simulink model "WorkstationModel_dynamicSequencing"  (R2015b)
settings: Solver=VariableStepDiscrete  StartTime=0.0  StopTime=1000  RelTol=1e-3
undefined symbols (not defined in the file): des
settings Model: Creator=tsprock3  LastModifiedBy=tsprock3
settings SolverCC: MaxConsecutiveZCs=10000
settings DataIOCC: InitialState=state  SaveFinalState=on  SaveFormat=Array
settings HardwareCC: ProdBitPerPointer=32  ProdLargestAtomicFloat=None  ProdIntDivRoundTo=Undefined  ProdEndianess=Unspecified  ProdWordSize=32  ProdHWDeviceType=32-bit Generic
settings GRTTargetCC: GeneratePreprocessorConditionals=Disable all
settings ConfigComp: CovModelRefEnable=Off

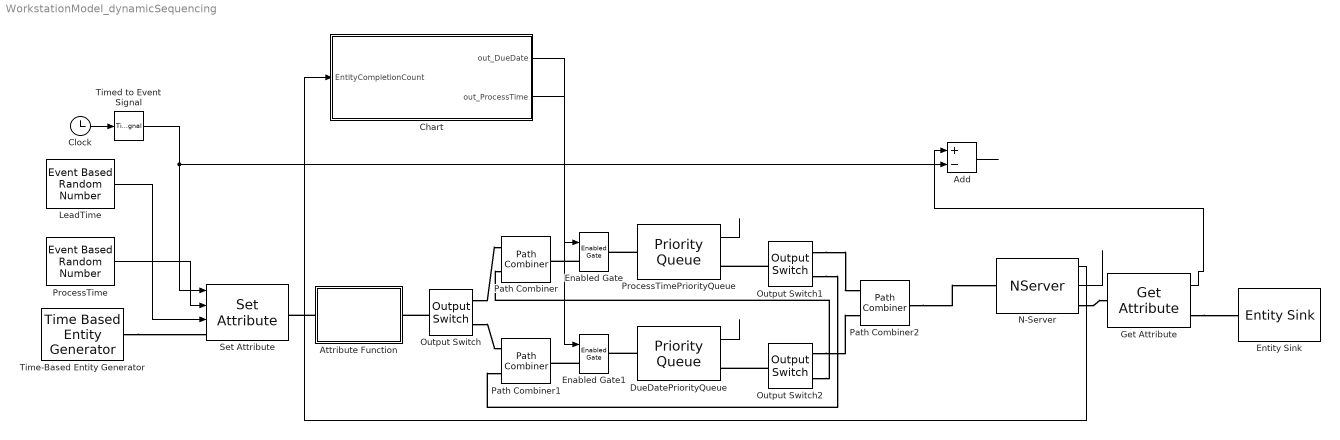
== system WorkstationModel_dynamicSequencing ==
  Add : Sum  Inputs=+-
  Attribute Function : Subsystem  LoadFcn=des.afb.attributefunction_support(gcb,'LoadFcn');  StartFcn=des.afb.attributefunction_support(gcb,'StartFcn');  mask(Attribute Function){OutputNamePrefix=out_}
      mask prompts: OutputNamePrefix "Prefix name"
      settings: CopyFcn=des.afb.attributefunction_support(gcb,'CopyFcn');  OpenFcn=des.afb.attributefunction_support(gcb,'OpenFcn');  ErrorFcn=des.afb.error_redirect
      mask Help: slhelp(gcbh)
      mask Display: image(des_iconLoad('attribFunction.jpg'),'center');
  Chart : Stateflow chart  TreatAsAtomicUnit=on
  Clock : Clock
  DueDatePriorityQueue : PriorityQueue  Capacity=inf  SortingAttributeName=DueDate  StatNumberInBlock=on
      settings: OutputPortMap=o1
  Enabled Gate : EnabledGate
  Enabled Gate1 : EnabledGate
  Entity Sink : EntitySink
  Get Attribute : GetAttribute  AttributeName=DueDate  EvaluatedDefaultAttributeValue={ []}
      settings: OutputPortMap=o1
  LeadTime : EventBasedRandomNumber  Distribution=Triangular  minTri=7  maxTri=15  modeTri=10  Seed=16319
  N-Server : NServer  NumberOfServers=4  ServiceTimeFrom=Attribute  AttributeName=ProcessTime  ServiceChange=Force complete  StatNumberDeparted=on  StatUtilization=on
      settings: OutputPortMap=o0,o5
  Output Switch : OutputSwitch  NumberOutputPorts=2
  Output Switch1 : OutputSwitch  NumberOutputPorts=2
  Output Switch2 : OutputSwitch  NumberOutputPorts=2
  Path Combiner : PathCombiner  NumberInputPorts=2
  Path Combiner1 : PathCombiner  NumberInputPorts=2
  Path Combiner2 : PathCombiner  NumberInputPorts=2
  ProcessTime : EventBasedRandomNumber  meanExp=4  Seed=19536
  ProcessTimePriorityQueue : PriorityQueue  Capacity=inf  SortingAttributeName=ProcessTime  StatNumberInBlock=on
      settings: OutputPortMap=o1
  Set Attribute : SetAttribute  AttributeName=StartTime|ProcessTime|LeadTime|DueDate  AttributeFrom=Signal port|Signal port|Signal port|Dialog  AttributeValue=1|1|1|1  AttributeTreatAsVector=1|1|1|1  EvaluatedAttributeValue={ [];[];[];1}
      settings: InputPortMap=u0,u1,u2
  Time-Based Entity Generator : TimeBasedEntityGenerator  EntityType=Standard
  Timed to Event Signal : TimedToEventSignal
  wires:
  ProcessTime/1 -> Set Attribute/2
  Clock/1 -> Timed to Event Signal/1
  Timed to Event Signal/1 -> Set Attribute/1, Add/2
  LeadTime/1 -> Set Attribute/3
  Get Attribute/1 -> Add/1
  Add/1 -> ?
  ProcessTimePriorityQueue/1 -> ?
  DueDatePriorityQueue/1 -> ?
  Chart/1(out_DueDate) -> Enabled Gate1/1
  Chart/2(out_ProcessTime) -> Enabled Gate/1
  N-Server/1 -> Chart/1(EntityCompletionCount)
  N-Server/2 -> ?
  connections:
  Time-Based Entity Generator/RConn1 -- Set Attribute/LConn1
  Attribute Function/LConn1 -- Set Attribute/RConn1
  N-Server/RConn1 -- Get Attribute/LConn1
  Get Attribute/RConn1 -- Entity Sink/LConn1
  Enabled Gate/LConn1 -- Path Combiner/RConn1
  ProcessTimePriorityQueue/LConn1 -- Enabled Gate/RConn1
  Output Switch/LConn1 -- Attribute Function/RConn1
  Output Switch/RConn1 -- Path Combiner/LConn1
  Enabled Gate1/LConn1 -- Path Combiner1/RConn1
  DueDatePriorityQueue/LConn1 -- Enabled Gate1/RConn1
  Output Switch/RConn2 -- Path Combiner1/LConn1
  Output Switch1/LConn1 -- ProcessTimePriorityQueue/RConn1
  Path Combiner2/RConn1 -- N-Server/LConn1
  Output Switch1/RConn1 -- Path Combiner2/LConn1
  Output Switch2/LConn1 -- DueDatePriorityQueue/RConn1
  Output Switch2/RConn1 -- Path Combiner2/LConn2
  Output Switch1/RConn2 -- Path Combiner1/LConn2
  Output Switch2/RConn2 -- Path Combiner/LConn2

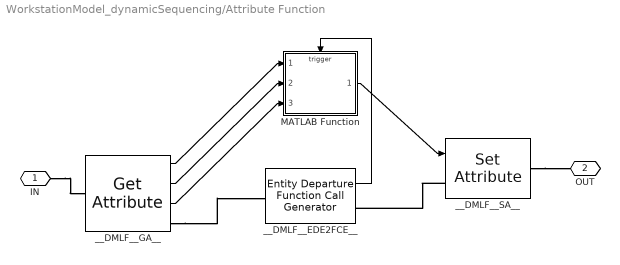
== system WorkstationModel_dynamicSequencing/Attribute Function ==
  MATLAB Function : MATLAB Function  TreatAsAtomicUnit=on
  __DMLF__EDE2FCE__ : EntityDepartureFunctionCallGenerator  TimingFunctionCallF1=Before entity departure  IsInsideAFB=on
  __DMLF__GA__ : GetAttribute  AttributeName=StartTime|LeadTime|DueDate  AttributeMissing=Error|Error|Error  AttributeDefaultValue=1|1|1  AttributeTreatAsVector=1|1|1  AttributeSendTiming=Before entity departure|Before entity departure|Before entity departure  EvaluatedDefaultAttributeValue={ [];[];[]}  IsInsideAFB=on
      settings: OutputPortMap=o1,o2,o3
  __DMLF__SA__ : SetAttribute  AttributeName=DueDate  AttributeFrom=Signal port  EvaluatedAttributeValue={ []}  IsInsideAFB=on
  IN : PMIOPort  Port=1  Side=Left
  OUT : PMIOPort  Port=2  Side=Right
  wires:
  __DMLF__EDE2FCE__/1 -> MATLAB Function/Trigger
  __DMLF__GA__/1 -> MATLAB Function/1(StartTime)
  __DMLF__GA__/2 -> MATLAB Function/2(LeadTime)
  __DMLF__GA__/3 -> MATLAB Function/3(DueDate)
  MATLAB Function/1(out_DueDate) -> __DMLF__SA__/1
  connections:
  __DMLF__SA__/LConn1 -- __DMLF__EDE2FCE__/RConn1
  __DMLF__GA__/RConn1 -- __DMLF__EDE2FCE__/LConn1
  IN/RConn1 -- __DMLF__GA__/LConn1
  __DMLF__SA__/RConn1 -- OUT/RConn1

== matlab function WorkstationModel_dynamicSequencing/Attribute Function/MATLAB Function ==
  data: StartTime input; out_DueDate output; LeadTime input; DueDate input
  events: trigger input FUNCTION_CALL_EVENT
function out_DueDate  = fcn(StartTime, LeadTime, DueDate)
%FCN    Access and modify attributes with MATLAB 
% 
out_DueDate = StartTime + LeadTime;

== stateflow chart WorkstationModel_dynamicSequencing/Chart ==
  state SequencingBehavior
    (history)
    state ProcessTimePriority
      en:
      out_DueDate = 0;
      out_ProcessTime = 1;
    state DueDatePriority
      en:
      out_DueDate = 1;
      out_ProcessTime = 0;
    DueDatePriority -> ProcessTimePriority : [mod(EntityCompletionCount,25) ==0]
    ProcessTimePriority -> DueDatePriority : [mod(EntityCompletionCount,25) ==0]
    (default) -> DueDatePriority
  (default) -> SequencingBehavior
  data: EntityCompletionCount input; out_DueDate output; out_ProcessTime output
